simulink model "PlantaPIL"  (R2022b)
settings: Solver=ode1  StartTime=0.0  StopTime=SIMULPARAM.T_end  FixedStep=SIMULPARAM.Ts  RelTol=1e-3  EnableMultiTasking=on
InitFcn:
  | System_Parameters;
StopFcn:
  | ShowResults;
undefined symbols (not defined in the file or in its folder): Bat_cell, C_fil, C_fil_0, ENV, IPM, Ki_current_bat, Ki_current_sc, Ki_d_cur, Ki_q_cur, Kp_current_bat, Kp_current_sc, Kp_d_cur, Kp_q_cur, Kp_voltage, Kp_Vveh, L_bat, L_sc, n_bat_par, n_bat_seri, n_sc_par, n_sc_seri, Nbat, Ninv, Nsc, P1_I, P_I, R1_on, R_on, Rth, SC_modul, SC_pack, u_dc_ref, VEH
libraries: esp32_device_config_lib x1, simulink x1
(part 2 of 2)

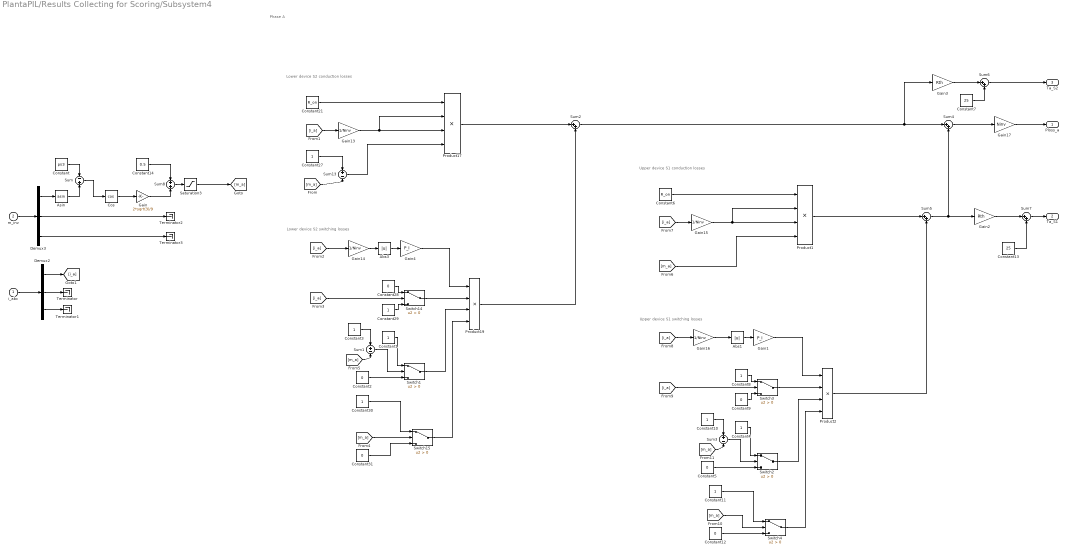
== system PlantaPIL/Results Collecting for Scoring/Subsystem4 ==
  note: Phase A
  note: Lower device S2 conduction losses
  note: Lower device S2 switching losses
  note: Upper device S1 conduction losses
  note: Upper device S1 switching losses
  i_abc : Inport
  m_inv : Inport  Port=2
  Abs1 : Abs  SaturateOnIntegerOverflow=off
  Abs3 : Abs  SaturateOnIntegerOverflow=off
  Asin : Trigonometry  Operator=asin
  Constant : Constant  Value=pi/3
  Constant{1,3..4,8,10..11,27,29..30} (9 alike) : Constant
  Constant{2,5,9,12,28,31} (6 alike) : Constant  Value=0
  Constant13 : Constant  Value=25
  Constant14 : Constant  Value=0.5
  Constant21 : Constant  Value=R_on
  Constant6 : Constant  Value=R_on
  Constant7 : Constant  Value=25
  Cos : Trigonometry  Operator=cos
  Demux2 : Demux  Outputs=3
  Demux3 : Demux  Outputs=3
  Gain : Gain  Gain=2*sqrt(3)/9
  Gain1 : Gain  Gain=P_I
  Gain{13..16} (4 alike) : Gain  Gain=1/Ninv
  Gain17 : Gain  Gain=Ninv
  Gain2 : Gain  Gain=Rth
  Gain3 : Gain  Gain=Rth
  Gain4 : Gain  Gain=P_I
  Product{1..2,17,19} (4 alike) : Product  Inputs=4
  Saturation3 : Saturate  UpperLimit=1  LowerLimit=0
  Sum : Sum  Inputs=-+
  Sum1 : Sum  Inputs=+-
  Sum13 : Sum  Inputs=+-
  Sum{2,4..7} (5 alike) : Sum  Inputs=|++
  Sum3 : Sum  Inputs=+-
  Sum8 : Sum
  Switch{1..4,14..15} (6 alike) : Switch  Criteria=u2 > Threshold  SaturateOnIntegerOverflow=off  InputSameDT=off
  Terminator{,1..3} (4 alike) : Terminator
  Ploss_a : Outport
  Ta_S1 : Outport  Port=2
  Ta_S2 : Outport  Port=3
  wires:
  i_abc/1 -> Demux2/1
  m_inv/1 -> Demux3/1
  Abs3/1 -> Gain4/1
  Constant21/1 -> Product17/1
  Constant28/1 -> Switch14/1
  Constant29/1 -> Switch14/3
  Gain4/1 -> Product19/1
  Constant31/1 -> Switch15/3
  Switch14/1 -> Product19/2
  Constant30/1 -> Switch15/1
  Demux2/1 -> [i_a]
  Demux2/2 -> Terminator/1
  Demux2/3 -> Terminator1/1
  Saturation3/1 -> [m_a]
  [m_a] -> Sum13/2
  Constant27/1 -> Sum13/1
  Sum13/1 -> Product17/4
  [i_a] -> Gain13/1
  [i_a] -> Gain14/1
  [i_a] -> Switch14/2
  [m_a] -> Switch15/2
  Constant1/1 -> Switch1/1
  Constant2/1 -> Switch1/3
  [m_a] -> Sum1/2
  Constant3/1 -> Sum1/1
  Sum1/1 -> Switch1/2
  Switch1/1 -> Product19/3
  Switch15/1 -> Product19/4
  Product17/1 -> Sum2/1
  Product19/1 -> Sum2/2
  Switch4/1 -> Product2/4
  [i_a] -> Gain16/1
  Sum3/1 -> Switch2/2
  [i_a] -> Gain15/1
  [i_a] -> Switch3/2
  Constant4/1 -> Switch2/1
  [m_a] -> Sum3/2
  Constant5/1 -> Switch2/3
  Constant11/1 -> Switch4/1
  Abs1/1 -> Gain1/1
  Switch3/1 -> Product2/2
  Constant9/1 -> Switch3/3
  Constant8/1 -> Switch3/1
  Switch2/1 -> Product2/3
  Gain1/1 -> Product2/1
  Product1/1 -> Sum5/1
  Constant12/1 -> Switch4/3
  [m_a] -> Switch4/2
  Constant10/1 -> Sum3/1
  Constant6/1 -> Product1/1
  Product2/1 -> Sum5/2
  [m_a] -> Product1/4
  Sum2/1 -> Gain3/1, Sum4/1
  Sum4/1 -> Gain17/1
  Gain13/1 -> Product17/2, Product17/3
  Gain14/1 -> Abs3/1
  Gain15/1 -> Product1/2, Product1/3
  Gain16/1 -> Abs1/1
  Gain17/1 -> Ploss_a/1
  Sum5/1 -> Gain2/1, Sum4/2
  Gain2/1 -> Sum7/1
  Constant13/1 -> Sum7/2
  Sum7/1 -> Ta_S1/1
  Gain3/1 -> Sum6/1
  Constant7/1 -> Sum6/2
  Sum6/1 -> Ta_S2/1
  Demux3/2 -> Terminator2/1
  Demux3/3 -> Terminator3/1
  Asin/1 -> Sum/2
  Constant/1 -> Sum/1
  Sum/1 -> Cos/1
  Cos/1 -> Gain/1
  Gain/1 -> Sum8/2
  Constant14/1 -> Sum8/1
  Sum8/1 -> Saturation3/1
  Demux3/1 -> Asin/1

== system PlantaPIL/Results Collecting for Scoring/Supercapacitor Branch Measurement ==
  u_sc : Outport  VectorParamsAs1DForOutWhenUnconnected=off
  i_sc : Outport  Port=2  VectorParamsAs1DForOutWhenUnconnected=off
  u_sc_modul : Outport  Port=3  VectorParamsAs1DForOutWhenUnconnected=off
  i_sc_modul : Outport  Port=4  VectorParamsAs1DForOutWhenUnconnected=off
  i_ch_sc : Outport  Port=5  VectorParamsAs1DForOutWhenUnconnected=off
  m_sc : Outport  Port=6  VectorParamsAs1DForOutWhenUnconnected=off
  i_ch_sc_ref : Outport  Port=7  VectorParamsAs1DForOutWhenUnconnected=off
  i_sc_ref : Outport  Port=8  VectorParamsAs1DForOutWhenUnconnected=off
  u_ch_sc_ref : Outport  Port=9  VectorParamsAs1DForOutWhenUnconnected=off
  SoC_SC : Outport  Port=10  VectorParamsAs1DForOutWhenUnconnected=off
  wires:
  [u_sc] -> u_sc/1
  [i_sc] -> i_sc/1
  [u_sc_modul] -> u_sc_modul/1
  [i_sc_modul] -> i_sc_modul/1
  [i_ch_sc] -> i_ch_sc/1
  [m_sc] -> m_sc/1
  [i_ch_sc_ref] -> i_ch_sc_ref/1
  [i_sc_ref] -> i_sc_ref/1
  [u_ch_sc_ref] -> u_ch_sc_ref/1
  [SoC_SC] -> SoC_SC/1

== system PlantaPIL/Results Collecting for Scoring/Vehicle Measurement ==
  Constant : Constant  Value=10^-4
  Product : Product  Inputs=3
  Sum : Sum  Inputs=+-
  Travel_dist : Outport  VectorParamsAs1DForOutWhenUnconnected=off
  u_dc : Outport  Port=2  VectorParamsAs1DForOutWhenUnconnected=off
  i_dc : Outport  Port=3  VectorParamsAs1DForOutWhenUnconnected=off
  v_veh : Outport  Port=4  VectorParamsAs1DForOutWhenUnconnected=off
  v_veh_ref : Outport  Port=5  VectorParamsAs1DForOutWhenUnconnected=off
  Potencia_Req : Outport  Port=6
  ErrorVelocidad : Outport  Port=7
  wires:
  [Travel_dist] -> Travel_dist/1
  [u_dc] -> u_dc/1
  [i_dc] -> i_dc/1
  [v_veh] -> v_veh/1
  [v_veh_ref] -> v_veh_ref/1
  [i_dc] -> Product/2
  [u_dc] -> Product/1
  Constant/1 -> Product/3
  Product/1 -> Potencia_Req/1
  [v_veh_ref] -> Sum/1
  Sum/1 -> ErrorVelocidad/1
  [v_veh] -> Sum/2

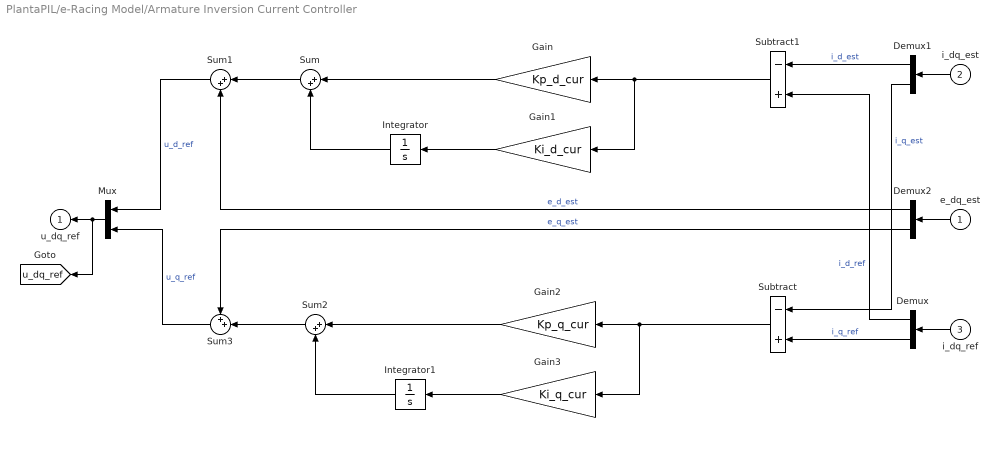
== system PlantaPIL/e-Racing Model/Armature Inversion Current Controller ==
  e_dq_est : Inport
  i_dq_est : Inport  Port=2
  i_dq_ref : Inport  Port=3
  Demux : Demux  Outputs=2
  Demux1 : Demux  Outputs=2
  Demux2 : Demux  Outputs=2
  Gain : Gain  Gain=Kp_d_cur
  Gain1 : Gain  Gain=Ki_d_cur
  Gain2 : Gain  Gain=Kp_q_cur
  Gain3 : Gain  Gain=Ki_q_cur
  Integrator : Integrator
  Integrator1 : Integrator
  Mux : Mux  Inputs=2
  Subtract : Sum  Inputs=-+
  Subtract1 : Sum  Inputs=-+
  Sum : Sum  Inputs=|++
  Sum1 : Sum  Inputs=|++
  Sum2 : Sum  Inputs=|++
  Sum3 : Sum  Inputs=++|
  u_dq_ref : Outport  InitialOutput=0  VectorParamsAs1DForOutWhenUnconnected=off
  tag scope: u_dq_ref=global
  wires:
  i_dq_ref/1 -> Demux/1
  i_dq_est/1 -> Demux1/1
  Demux/2 -> Subtract/2  "i_q_ref"
  Demux/1 -> Subtract1/2  "i_d_ref"
  Demux1/2 -> Subtract/1  "i_q_est"
  Demux1/1 -> Subtract1/1  "i_d_est"
  e_dq_est/1 -> Demux2/1
  Gain1/1 -> Integrator/1
  Gain/1 -> Sum/1
  Integrator/1 -> Sum/2
  Sum/1 -> Sum1/1
  Demux2/1 -> Sum1/2  "e_d_est"
  Subtract1/1 -> Gain1/1, Gain/1
  Mux/1 -> [u_dq_ref], u_dq_ref/1
  Sum1/1 -> Mux/1  "u_d_ref"
  Gain3/1 -> Integrator1/1
  Gain2/1 -> Sum2/1
  Integrator1/1 -> Sum2/2
  Sum3/1 -> Mux/2  "u_q_ref"
  Subtract/1 -> Gain3/1, Gain2/1
  Sum2/1 -> Sum3/2
  Demux2/2 -> Sum3/1  "e_q_est"

== system PlantaPIL/e-Racing Model/Chasis ==
  F_trac : Inport
  F_res : Inport  Port=2
  Gain : Gain  Gain=1/VEH.Mass
  Integrator : Integrator
  Sum : Sum  Inputs=|+-
  v_veh : Outport  InitialOutput=0  VectorParamsAs1DForOutWhenUnconnected=off
  "v_veh  " : Outport  Port=2  InitialOutput=0  VectorParamsAs1DForOutWhenUnconnected=off
  wires:
  F_trac/1 -> Sum/1
  F_res/1 -> Sum/2
  Sum/1 -> Gain/1
  Gain/1 -> Integrator/1
  Integrator/1 -> "v_veh  "/1, v_veh/1

== system PlantaPIL/e-Racing Model/Chasis Inversion  ==
  Fenv_meas : Inport
  Vveh_meas : Inport  Port=2
  Vveh_ref : Inport  Port=3
  Add : Sum
  Gain : Gain  Gain=Kp_Vveh
  Subtract : Sum  Inputs=-+
  Ftrac_ref : Outport  InitialOutput=0  VectorParamsAs1DForOutWhenUnconnected=off
  wires:
  Vveh_ref/1 -> Subtract/2
  Vveh_meas/1 -> Subtract/1
  Subtract/1 -> Gain/1
  Fenv_meas/1 -> Add/1
  Gain/1 -> Add/2
  Add/1 -> Ftrac_ref/1

== system PlantaPIL/e-Racing Model/E//M Conversion Inversion ==
  T_e_ref : Inport
  i_d_ref : Inport  Port=2
  Add : Sum
  Constant : Constant  Value=IPM.psi
  Divide : Product  Inputs=/*
  Gain : Gain  Gain=4/(3*IPM.p)
  Gain6 : Gain  Gain=IPM.L_d-IPM.L_q
  Memory : Memory
  Mux : Mux  Inputs=2
  i_dq_ref : Outport  InitialOutput=0  VectorParamsAs1DForOutWhenUnconnected=off
  tag scope: i_q_ref=global
  wires:
  Mux/1 -> i_dq_ref/1
  T_e_ref/1 -> Gain/1
  Gain/1 -> Divide/2
  Gain6/1 -> Add/1
  Constant/1 -> Add/2
  Add/1 -> Divide/1
  Divide/1 -> [i_q_ref], Mux/2  "i_q_ref"
  i_d_ref/1 -> Memory/1  "i_d_ref"
  Memory/1 -> Mux/1, Gain6/1

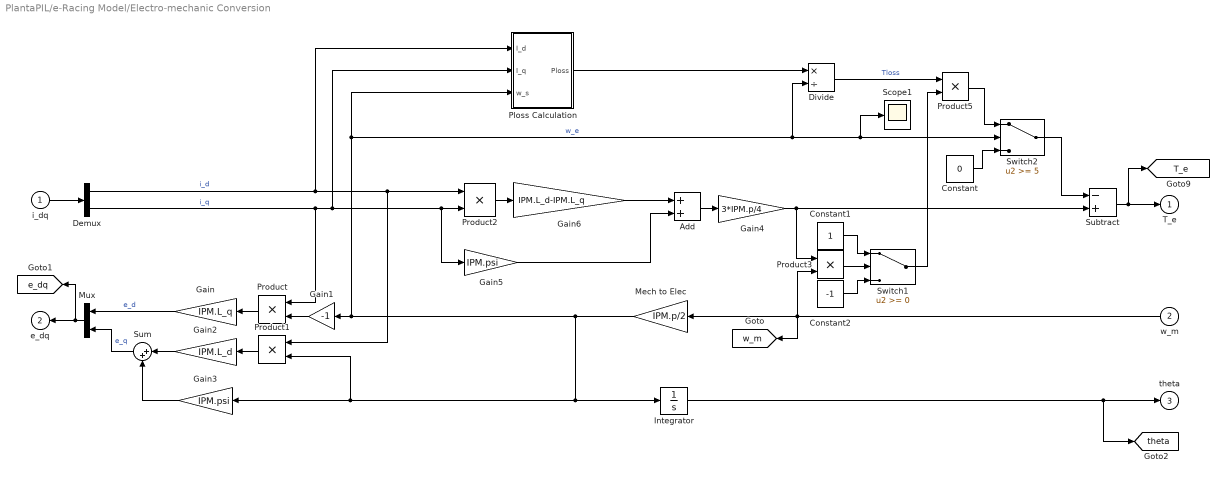
== system PlantaPIL/e-Racing Model/Electro-mechanic Conversion ==
  i_dq : Inport
  w_m : Inport  Port=2
  Add : Sum
  Constant : Constant  Value=0
  Constant1 : Constant
  Constant2 : Constant  Value=-1
  Demux : Demux  Outputs=2
  Divide : Product  Inputs=*/
  Gain : Gain  Gain=IPM.L_q
  Gain1 : Gain  Gain=-1
  Gain2 : Gain  Gain=IPM.L_d
  Gain3 : Gain  Gain=IPM.psi
  Gain4 : Gain  Gain=3*IPM.p/4
  Gain5 : Gain  Gain=IPM.psi
  Gain6 : Gain  Gain=IPM.L_d-IPM.L_q
  Integrator : Integrator
  Mech to Elec : Gain  Gain=IPM.p/2
  Mux : Mux  Inputs=2
  Ploss Calculation : Subsystem
  Product{,1..3,5} (5 alike) : Product
  Scope1 : Scope
  Subtract : Sum  Inputs=-+
  Sum : Sum  Inputs=|++
  Switch1 : Switch  SaturateOnIntegerOverflow=off  InputSameDT=off
  Switch2 : Switch  Threshold=5  SaturateOnIntegerOverflow=off  InputSameDT=off
  T_e : Outport  VectorParamsAs1DForOutWhenUnconnected=off
  e_dq : Outport  Port=2  VectorParamsAs1DForOutWhenUnconnected=off
  theta : Outport  Port=3  VectorParamsAs1DForOutWhenUnconnected=off
  tag scope: T_e=global, e_dq=global, theta=global, w_m=global
  wires:
  Mux/1 -> [e_dq], e_dq/1
  i_dq/1 -> Demux/1
  Add/1 -> Gain4/1
  Gain3/1 -> Sum/2
  Product2/1 -> Gain6/1
  Switch1/1 -> Product5/2
  Ploss Calculation/1(Ploss) -> Divide/1
  Product1/1 -> Gain2/1
  Demux/2 -> Product/1, Gain5/1, Product2/2, Ploss Calculation/2(I_q)  "i_q"
  Mech to Elec/1 -> Integrator/1, Gain3/1, Product1/2, Scope1/1, Switch2/2, Divide/2, Ploss Calculation/3(w_s), Gain1/1  "w_e"
  Gain2/1 -> Sum/1
  Constant1/1 -> Switch1/1
  Product/1 -> Gain/1
  Switch2/1 -> Subtract/1
  Gain6/1 -> Add/1
  Gain5/1 -> Add/2
  Product5/1 -> Switch2/1
  Product3/1 -> Switch1/2
  w_m/1 -> [w_m], Product3/2, Mech to Elec/1
  Sum/1 -> Mux/2  "e_q"
  Gain/1 -> Mux/1  "e_d"
  Demux/1 -> Ploss Calculation/1(I_d), Product2/1, Product1/1  "i_d"
  Integrator/1 -> [theta], theta/1
  Constant2/1 -> Switch1/3
  Divide/1 -> Product5/1  "Tloss"
  Gain1/1 -> Product/2
  Constant/1 -> Switch2/3
  Gain4/1 -> Product3/1, Subtract/2
  Subtract/1 -> [T_e], T_e/1

== system PlantaPIL/e-Racing Model/Environment ==
  v_veh : Inport
  Abs : Abs  SaturateOnIntegerOverflow=off
  Add : Sum
  Fcn : Fcn  Expr=ENV.air*(u(1)+ENV.v_wind)^2+u(2)
  Gain : Gain  Gain=5
  Manual Switch : ManualSwitch
  Mux : Mux  Inputs=2
  Product : Product  RndMeth=Zero
  Saturation : Saturate  UpperLimit=1  LowerLimit=0
  pente de 0% : Constant  Value=ENV.slope0
  pente de 10% : Constant  Value=ENV.slope10
  pente de 10%1 : Constant  Value=ENV.roll
  F_res : Outport  InitialOutput=0  VectorParamsAs1DForOutWhenUnconnected=off
  wires:
  Gain/1 -> Saturation/1
  Saturation/1 -> Product/1
  Abs/1 -> Gain/1
  Mux/1 -> Fcn/1
  v_veh/1 -> Mux/1, Abs/1
  Add/1 -> F_res/1
  pente de 10%1/1 -> Product/2
  Product/1 -> Add/2
  Fcn/1 -> Add/1
  Manual Switch/1 -> Mux/2
  pente de 0%/1 -> Manual Switch/1
  pente de 10%/1 -> Manual Switch/2

== system PlantaPIL/e-Racing Model/Gearbox ==
  T_e : Inport
  W_gear : Inport  Port=2
  Gain : Gain  Gain=VEH.k_gear
  Gain1 : Gain  Gain=VEH.TransEff
  Gain2 : Gain  Gain=1/VEH.TransEff
  Gain3 : Gain  Gain=VEH.k_gear
  Product : Product
  Switch : Switch  Criteria=u2 > Threshold  SaturateOnIntegerOverflow=off  InputSameDT=off
  T_gear : Outport  InitialOutput=0  VectorParamsAs1DForOutWhenUnconnected=off
  w_m : Outport  Port=2  InitialOutput=0  VectorParamsAs1DForOutWhenUnconnected=off
  wires:
  Product/1 -> Switch/2
  T_e/1 -> Gain2/1, Gain1/1, Product/1
  W_gear/1 -> Gain/1
  Gain/1 -> Product/2, w_m/1
  Gain1/1 -> Switch/1
  Gain2/1 -> Switch/3
  Switch/1 -> Gain3/1
  Gain3/1 -> T_gear/1

== system PlantaPIL/e-Racing Model/Gearbox Inversion ==
  T_gear_ref : Inport
  Gain : Gain  Gain=1/VEH.k_gear
  T_e_ref : Outport  InitialOutput=0  VectorParamsAs1DForOutWhenUnconnected=off
  tag scope: T_e_ref=global
  wires:
  Gain/1 -> [T_e_ref], T_e_ref/1
  T_gear_ref/1 -> Gain/1

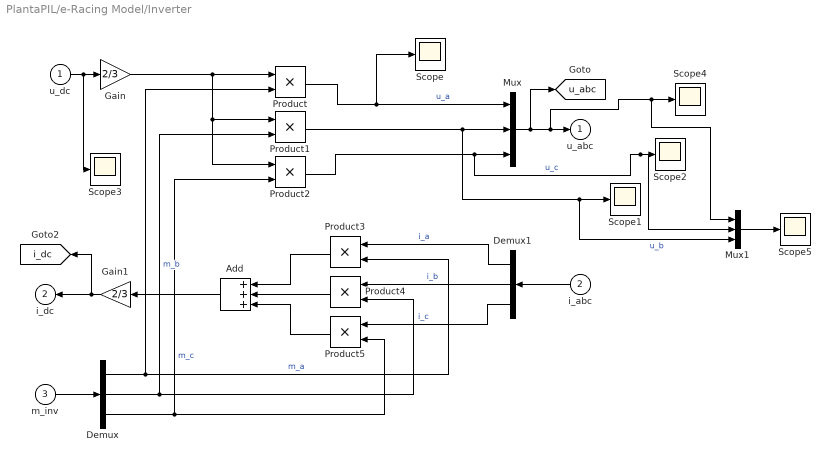
== system PlantaPIL/e-Racing Model/Inverter ==
  u_dc : Inport
  i_abc : Inport  Port=2
  m_inv : Inport  Port=3
  Add : Sum  Inputs=3
  Demux : Demux  Outputs=3
  Demux1 : Demux  Outputs=3
  Gain : Gain  Gain=2/3
  Gain1 : Gain  Gain=2/3
  Mux : Mux  Inputs=3
  Mux1 : Mux  Inputs=3
  Product{,1..5} (6 alike) : Product
  Scope{,1..5} (6 alike) : Scope
  u_abc : Outport  InitialOutput=0  VectorParamsAs1DForOutWhenUnconnected=off
  i_dc : Outport  Port=2  InitialOutput=0  VectorParamsAs1DForOutWhenUnconnected=off
  tag scope: i_dc=global, u_abc=global
  wires:
  Mux/1 -> [u_abc], Mux1/1, Scope4/1, u_abc/1
  m_inv/1 -> Demux/1
  u_dc/1 -> Scope3/1, Gain/1
  Gain/1 -> Product2/1, Product1/1, Product/1
  Demux/1 -> Product/2, Product3/2  "m_a"
  Demux/2 -> Product1/2, Product4/2  "m_b"
  Demux/3 -> Product5/2, Product2/2  "m_c"
  Product/1 -> Scope/1, Mux/1  "u_a"
  Product1/1 -> Mux1/3, Scope1/1, Mux/2  "u_b"
  Product2/1 -> Mux1/2, Scope2/1, Mux/3  "u_c"
  i_abc/1 -> Demux1/1
  Demux1/1 -> Product3/1  "i_a"
  Demux1/2 -> Product4/1  "i_b"
  Demux1/3 -> Product5/1  "i_c"
  Product3/1 -> Add/1
  Product4/1 -> Add/2
  Product5/1 -> Add/3
  Add/1 -> Gain1/1
  Gain1/1 -> [i_dc], i_dc/1
  Mux1/1 -> Scope5/1

== system PlantaPIL/e-Racing Model/Inverter Inversion ==
  "u_dc_meas " : Inport
  u_abc_ref : Inport  Port=2
  Divide : Product  Inputs=*/
  Gain : Gain  Gain=0.5
  Saturation : Saturate  UpperLimit=1  LowerLimit=-1
  m_inv : Outport  InitialOutput=0  VectorParamsAs1DForOutWhenUnconnected=off
  tag scope: m_inv=global
  wires:
  Divide/1 -> Saturation/1
  u_abc_ref/1 -> Divide/1
  "u_dc_meas "/1 -> Gain/1
  Saturation/1 -> [m_inv], m_inv/1
  Gain/1 -> Divide/2

== system PlantaPIL/e-Racing Model/Motor Winding ==
  u_dq : Inport
  e_dq : Inport  Port=2
  Demux : Demux  Outputs=2
  Demux1 : Demux  Outputs=2
  Mux : Mux  Inputs=2
  Subtract : Sum  Inputs=+-
  Subtract1 : Sum  Inputs=+-
  Transfer Fcn : TransferFcn  Denominator=[IPM.L_d IPM.R_s]
  Transfer Fcn1 : TransferFcn  Denominator=[IPM.L_q IPM.R_s]
  i_dq : Outport  InitialOutput=0  VectorParamsAs1DForOutWhenUnconnected=off
  "i_dq " : Outport  Port=2  InitialOutput=0  VectorParamsAs1DForOutWhenUnconnected=off
  tag scope: i_dq=global
  wires:
  u_dq/1 -> Demux/1
  e_dq/1 -> Demux1/1
  Mux/1 -> [i_dq], "i_dq "/1, i_dq/1
  Demux/1 -> Subtract/1  "u_d"
  Demux1/1 -> Subtract/2  "e_d"
  Subtract/1 -> Transfer Fcn/1
  Transfer Fcn/1 -> Mux/1  "i_d"
  Subtract1/1 -> Transfer Fcn1/1
  Demux/2 -> Subtract1/1  "u_q"
  Demux1/2 -> Subtract1/2  "e_q"
  Transfer Fcn1/1 -> Mux/2  "i_q"

== system PlantaPIL/e-Racing Model/Wheel ==
  T_gear : Inport
  v_veh : Inport  Port=2
  Gain : Gain  Gain=1/VEH.WheelRad
  Gain1 : Gain  Gain=1/VEH.WheelRad
  F_trac : Outport  InitialOutput=0  VectorParamsAs1DForOutWhenUnconnected=off
  W_gear : Outport  Port=2  InitialOutput=0  VectorParamsAs1DForOutWhenUnconnected=off
  wires:
  T_gear/1 -> Gain/1
  Gain/1 -> F_trac/1
  Gain1/1 -> W_gear/1
  v_veh/1 -> Gain1/1

== system PlantaPIL/e-Racing Model/Wheel Inversion  ==
  Ftrac_ref : Inport
  Gain : Gain  Gain=VEH.WheelRad
  Tgear_ref : Outport  InitialOutput=0  VectorParamsAs1DForOutWhenUnconnected=off
  wires:
  Ftrac_ref/1 -> Gain/1
  Gain/1 -> Tgear_ref/1

== system PlantaPIL/e-Racing Model/abc//dq ==
  u_abc : Inport
  i_dq : Inport  Port=2
  theta : Inport  Port=3
  Inversed Park Transformation : Subsystem
  Park Transformation : Subsystem
  Product : Product  Multiplication=Matrix(*)
  Product1 : Product  Multiplication=Matrix(*)
  Scope{,1..3} (4 alike) : Scope
  u_dq : Outport  InitialOutput=0  VectorParamsAs1DForOutWhenUnconnected=off
  i_abc : Outport  Port=2  InitialOutput=0  VectorParamsAs1DForOutWhenUnconnected=off
  tag scope: i_abc=global, u_dq=global
  wires:
  theta/1 -> Inversed Park Transformation/1(Theta), Park Transformation/1(Theta)
  Product/1 -> Scope1/1, [u_dq], u_dq/1  "dq_value"
  Park Transformation/1(Matrix Out) -> Product/1
  u_abc/1 -> Scope/1, Product/2  "abc_value"
  Inversed Park Transformation/1(Matrix Out) -> Product1/1
  i_dq/1 -> Scope2/1, Product1/2  "dq_value"
  Product1/1 -> Scope3/1, [i_abc], i_abc/1  "abc_value"

== system PlantaPIL/e-Racing Model/dq//abc ==
  theta_meas : Inport
  u_dq_ref : Inport  Port=2
  Inversed Park Transformation : Subsystem
  Product1 : Product  Multiplication=Matrix(*)
  u_abc_ref : Outport  InitialOutput=0  VectorParamsAs1DForOutWhenUnconnected=off
  tag scope: u_abc_ref=global
  wires:
  Inversed Park Transformation/1(Matrix Out) -> Product1/1
  Product1/1 -> [u_abc_ref], u_abc_ref/1  "abc_value"
  u_dq_ref/1 -> Product1/2  "dq_value"
  theta_meas/1 -> Inversed Park Transformation/1(Theta)

== system PlantaPIL/DC-bus Inversion/SC Limitation/Limitation transition ==
  i_dc_meas : Inport
  i_bat_ref_cal : Inport  Port=2
  u_sc_meas : Inport  Port=3
  1-D Lookup Table : Lookup_n-D  NumberOfTableDimensions=1  BreakpointsForDimension1=[SC_pack.U_min SC_pack.U_hi SC_pack.U_max]  Table=[0 0 1]  InternalRulePriority=Speed  RndMeth=Simplest
  1-D Lookup Table1 : Lookup_n-D  NumberOfTableDimensions=1  BreakpointsForDimension1=[SC_pack.U_min SC_pack.U_low SC_pack.U_max]  Table=[1 0 0]  InternalRulePriority=Speed  RndMeth=Simplest
  Add1 : Sum  Inputs=+-
  Switch1 : Switch  SaturateOnIntegerOverflow=off  InputSameDT=off
  k_d : Outport  VectorParamsAs1DForOutWhenUnconnected=off
  wires:
  1-D Lookup Table/1 -> Switch1/3
  u_sc_meas/1 -> 1-D Lookup Table1/1, 1-D Lookup Table/1
  Add1/1 -> Switch1/2
  Switch1/1 -> k_d/1
  i_dc_meas/1 -> Add1/1
  i_bat_ref_cal/1 -> Add1/2
  1-D Lookup Table1/1 -> Switch1/1

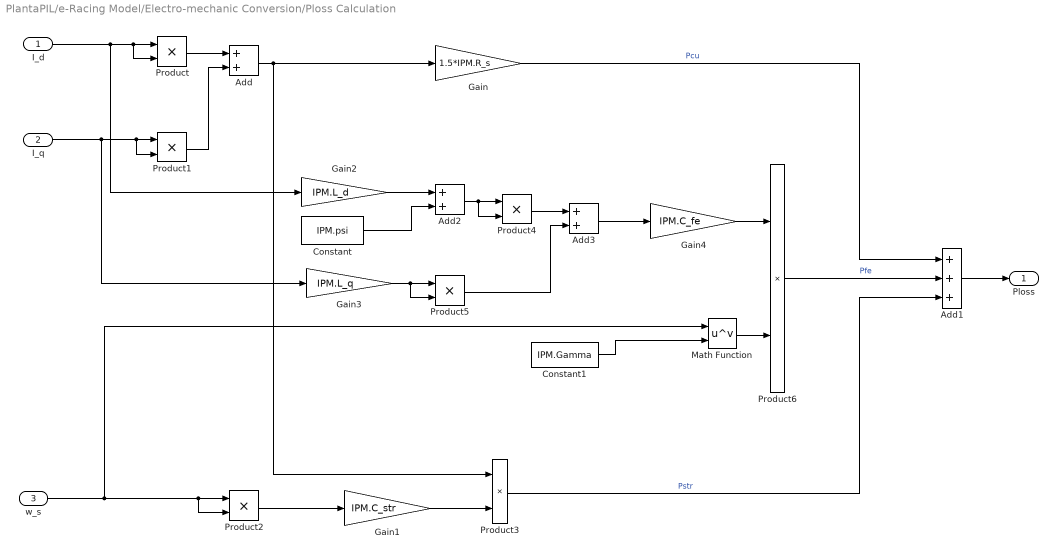
== system PlantaPIL/e-Racing Model/Electro-mechanic Conversion/Ploss Calculation ==
  I_d : Inport
  I_q : Inport  Port=2
  w_s : Inport  Port=3
  Add : Sum
  Add1 : Sum  Inputs=+++
  Add2 : Sum
  Add3 : Sum
  Constant : Constant  Value=IPM.psi
  Constant1 : Constant  Value=IPM.Gamma
  Gain : Gain  Gain=1.5*IPM.R_s
  Gain1 : Gain  Gain=IPM.C_str
  Gain2 : Gain  Gain=IPM.L_d
  Gain3 : Gain  Gain=IPM.L_q
  Gain4 : Gain  Gain=IPM.C_fe
  Math Function : Math  Operator=pow
  Product{,1..6} (7 alike) : Product
  Ploss : Outport
  wires:
  I_d/1 -> Gain2/1, Product/2, Product/1
  I_q/1 -> Gain3/1, Product1/2, Product1/1
  Product/1 -> Add/1
  Product1/1 -> Add/2
  Add/1 -> Gain/1, Product3/1
  w_s/1 -> Math Function/1, Product2/2, Product2/1
  Product2/1 -> Gain1/1
  Gain1/1 -> Product3/2
  Add1/1 -> Ploss/1
  Product3/1 -> Add1/3  "Pstr"
  Gain/1 -> Add1/1  "Pcu"
  Gain2/1 -> Add2/1
  Constant/1 -> Add2/2
  Add2/1 -> Product4/2, Product4/1
  Gain3/1 -> Product5/2, Product5/1
  Product4/1 -> Add3/1
  Product5/1 -> Add3/2
  Add3/1 -> Gain4/1
  Constant1/1 -> Math Function/2
  Gain4/1 -> Product6/1
  Math Function/1 -> Product6/2
  Product6/1 -> Add1/2  "Pfe"

== system PlantaPIL/e-Racing Model/abc//dq/Inversed Park Transformation ==
  Theta : Inport
  Cos : Trigonometry  Operator=cos
  Gain : Gain  Gain=-1
  Gain2 : Gain  Gain=[1 0; -1/2 sqrt(3)/2; -1/2 -sqrt(3)/2]  Multiplication=Matrix(K*u)
  Matrix Concatenate : Concatenate  Mode=Multidimensional array
  Mux : Mux  Inputs=2
  Mux1 : Mux  Inputs=2
  Sin : Trigonometry
  Transpose : Math  Operator=transpose  SignedPower=on
  Transpose1 : Math  Operator=transpose  SignedPower=on
  Matrix Out : Outport  VectorParamsAs1DForOutWhenUnconnected=off
  wires:
  Transpose1/1 -> Matrix Concatenate/2
  Transpose/1 -> Matrix Concatenate/1
  Matrix Concatenate/1 -> Gain2/1
  Gain2/1 -> Matrix Out/1
  Mux1/1 -> Transpose1/1
  Mux/1 -> Transpose/1
  Theta/1 -> Cos/1, Sin/1
  Cos/1 -> Mux1/2, Mux/1
  Gain/1 -> Mux/2
  Sin/1 -> Mux1/1, Gain/1

== system PlantaPIL/e-Racing Model/abc//dq/Park Transformation ==
  Theta : Inport
  Cos : Trigonometry  Operator=cos
  Gain : Gain  Gain=-1
  Gain1 : Gain  Gain=2/3
  Gain2 : Gain  Gain=[1 -1/2 -1/2; 0 sqrt(3)/2 -sqrt(3)/2]  Multiplication=Matrix(u*K)
  Matrix Concatenate : Concatenate  Mode=Multidimensional array
  Mux : Mux  Inputs=2
  Mux1 : Mux  Inputs=2
  Sin : Trigonometry
  Transpose : Math  Operator=transpose  SignedPower=on
  Transpose1 : Math  Operator=transpose  SignedPower=on
  Matrix Out : Outport  VectorParamsAs1DForOutWhenUnconnected=off
  wires:
  Theta/1 -> Sin/1, Cos/1
  Cos/1 -> Mux1/2, Mux/1
  Sin/1 -> Mux/2, Gain/1
  Gain/1 -> Mux1/1
  Mux/1 -> Transpose/1
  Mux1/1 -> Transpose1/1
  Gain1/1 -> Matrix Out/1
  Matrix Concatenate/1 -> Gain2/1
  Gain2/1 -> Gain1/1
  Transpose/1 -> Matrix Concatenate/1
  Transpose1/1 -> Matrix Concatenate/2

== system PlantaPIL/e-Racing Model/dq//abc/Inversed Park Transformation ==
  Theta : Inport
  Cos : Trigonometry  Operator=cos
  Gain : Gain  Gain=-1
  Gain2 : Gain  Gain=[1 0; -1/2 sqrt(3)/2; -1/2 -sqrt(3)/2]  Multiplication=Matrix(K*u)
  Matrix Concatenate : Concatenate  Mode=Multidimensional array
  Mux : Mux  Inputs=2
  Mux1 : Mux  Inputs=2
  Sin : Trigonometry
  Transpose : Math  Operator=transpose  SignedPower=on
  Transpose1 : Math  Operator=transpose  SignedPower=on
  Matrix Out : Outport  VectorParamsAs1DForOutWhenUnconnected=off
  wires:
  Transpose1/1 -> Matrix Concatenate/2
  Transpose/1 -> Matrix Concatenate/1
  Matrix Concatenate/1 -> Gain2/1
  Gain2/1 -> Matrix Out/1
  Mux1/1 -> Transpose1/1
  Mux/1 -> Transpose/1
  Theta/1 -> Cos/1, Sin/1
  Cos/1 -> Mux1/2, Mux/1
  Gain/1 -> Mux/2
  Sin/1 -> Mux1/1, Gain/1
